simulink model "model"  (R2022b)
settings: Solver=VariableStepAuto  StartTime=0.0  StopTime=10.0  RelTol=1e-3
values from neighbouring files (symbols this model uses):
  A = [-4.979 0 0.036 3.01 ... (first row only)    [matricies.m]
  B = [8.584 ... (first row only)    [matricies.m]
undefined symbols (not defined in the file or in its folder): Humusoft, kalmf, MF624
libraries: sldrtlib x3, simulink x1
settings Model: Creator=efrem  LastModifiedBy=126893
settings DebuggingCC: UnconnectedInputMsg=warning  UnconnectedOutputMsg=warning  UnconnectedLineMsg=warning
settings ModelReferenceCC: EnableRefExpFcnMdlSchedulingChecks=on
settings RTWCC: DLArmComputeVersion=19.05

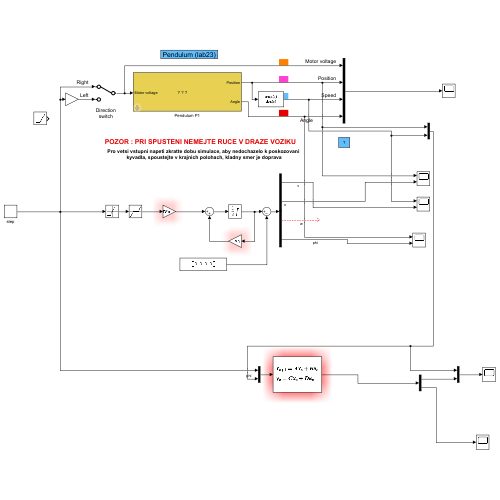
[thumbnail: Simulink's stored preview of the top-level diagram]
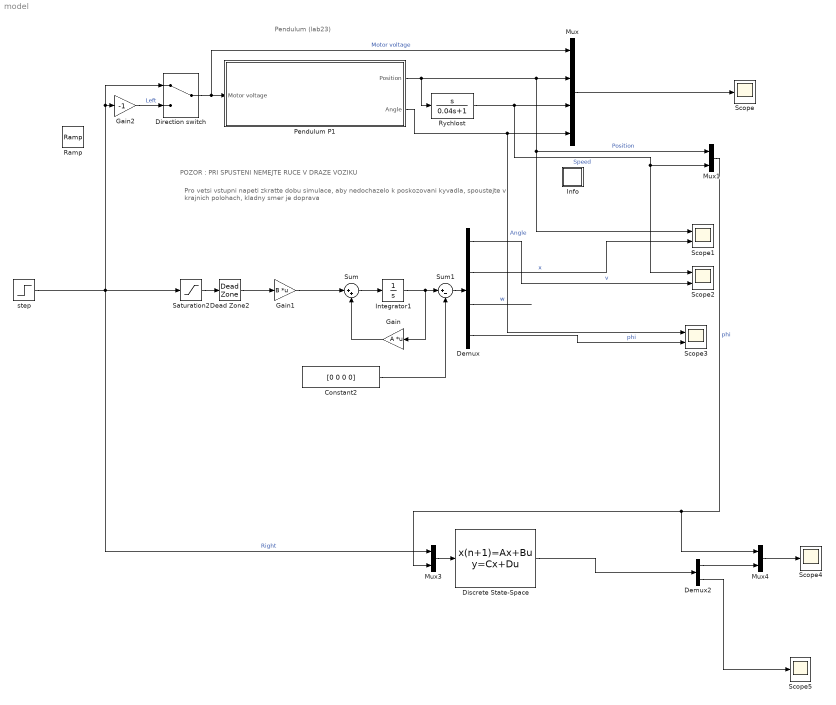
== system model ==
  note: POZOR : PRI SPUSTENI NEMEJTE RUCE V DRAZE VOZIKU
  note: Pro vetsi vstupni napeti zkratte dobu simulace, aby nedochazelo k poskozovani
      |  kyvadla, spoustejte v krajnich polohach, kladny smer je doprava
  note: Pendulum (lab23)
  Constant2 : Constant  Value=[0 0 0 0]
  Dead Zone2 : DeadZone  LowerValue=-0.11  UpperValue=0.11
  Demux : Demux
      settings: DisplayOption=none
  Demux2 : Demux  Outputs=[1,2]
  Direction switch : ManualSwitch
  Discrete State-Space : DiscreteStateSpace  A=kalmf.A  B=kalmf.B  C=kalmf.C  D=kalmf.D  InitialCondition=[0.2,0]  SampleTime=kalmf.Ts
  Gain : Gain  Gain=A  Multiplication=Matrix(K*u)
  Gain1 : Gain  Gain=B  Multiplication=Matrix(K*u)
  Gain2 : Gain  Gain=-1
  Info : Subsystem
      mask Display: disp('?')
  Integrator1 : Integrator  InitialCondition=[0,0,0,0]  LimitOutput=on  UpperSaturationLimit=[inf, 0.35, inf, inf]  LowerSaturationLimit=-[inf, 0.35, inf, inf]
  Mux : Mux
  Mux1 : Mux  Inputs=2
  Mux3 : Mux  Inputs=2
  Mux4 : Mux  Inputs=2
  Pendulum P1 : Subsystem  InitFcn=warning off;  mask(Pendulum P1 in laboratory K23){Ts=0.001}
      mask prompts: Ts "Sampling time  {Ts = 0.001 s;   0.001 - 0.01 s}"
      mask help: Pendulum P1 in laboratory K23 - Real Time Communication
      mask Help:
      | Servo AMIRA S1, S4 in laboratory K23, K26 - Real Time Communication. <br><br>
      | 
      | This is a model of the Servomechanism, which is composed of two identical motors (motor and generator) connected together with solid motor shaft. First motor is used as a generator - it can be used to simulation of a varying  moment of inertia. The second motor takes control of the rotational speed of the servomechanism or the angle of turning of the motor shaft.<br>
      | 
      | There are two inputs and three outputs in the model. Inputs are voltages of generator and motor.
      | Outputs are speed of the servomechanism, the angle of turning of the motor shaft and current of the motor.<br><br>
      | In Simulink, the signals are normalized.
      mask Display: image(imread('P1pic.tif'))
  Ramp : simulink/Sources/Ramp  slope=1  start=0  InitialOutput=0
  Rychlost : TransferFcn  Numerator=[1 0]  Denominator=[0.04 1]
  Saturation2 : Saturate  UpperLimit=1  LowerLimit=-1
  Scope : Scope
  Scope1 : Scope  NumInputPorts=2
  Scope2 : Scope  NumInputPorts=2
  Scope3 : Scope  NumInputPorts=2
  Scope4 : Scope
  Scope5 : Scope
  Sum : Sum  Inputs=|++
  Sum1 : Sum  Inputs=|+-
  step : Step  After=0.2  SampleTime=0
  wires:
  Gain1/1 -> Sum/1
  Dead Zone2/1 -> Gain1/1
  Sum/1 -> Integrator1/1
  Gain/1 -> Sum/2
  Demux/2 -> Scope1/2  "x"
  Demux/1 -> Scope2/2  "v"
  Integrator1/1 -> Gain/1, Sum1/1
  Saturation2/1 -> Dead Zone2/1
  Sum1/1 -> Demux/1
  Constant2/1 -> Sum1/2
  Demux/3 -> ?  "w"
  Demux/4 -> Scope3/2  "phi"
  Direction switch/1 -> Pendulum P1/1(Motor voltage), Mux/1  "Motor voltage"
  Rychlost/1 -> Mux1/2, Scope2/1, Mux/3  "Speed"
  Pendulum P1/2(Angle) -> Scope3/1, Mux/4  "Angle"
  Gain2/1 -> Direction switch/2  "Left"
  Pendulum P1/1(Position) -> Scope1/1, Mux1/1, Mux/2, Rychlost/1  "Position"
  step/1 -> Saturation2/1, Mux3/1, Direction switch/1, Gain2/1  "Right"
  Mux/1 -> Scope/1
  Demux2/1 -> Mux4/2
  Discrete State-Space/1 -> Demux2/1
  Demux2/2 -> Scope5/1
  Mux4/1 -> Scope4/1
  Mux3/1 -> Discrete State-Space/1
  Mux1/1 -> Mux4/1, Mux3/2  "phi"

== system model/Info ==
  note: Urceno pro mereni prechodovych charakteristik realneho systemu inverzni kyvadlo.
      |  Periodu vzorkovani Ts volte v rozsahu 0.0005 s < Ts < 0.001 s  (dop. Ts = 0.001 s).
  note: Vozik presunte do leve krajni polohy. Po spusteni simulace dojede k prave krajni
      | poloze. Presunte jej ke koncovemu spinaci a zmente znamenko zesileni. Vozik
      | se vrati do vychozi polohy. Pri vetsim vstupnim napeti zkratte dobu simulace!!!
  note: Umisteni voziku
  note: Merena data jsou ukladana po radcich do matice ty v pracovnim prostoru Matlabu.
      | Prvni sloupec matice ty predstavuje cas a dalsi pak jednotlive promenne v poradi
      | vstupu do bloku multiplexoru osciloskopu. Krome toho je jeste k dispozici samotny
      | vektor casu tout. Prubehy velicin zobrazite napr. prikazem: plot(ty(:,1),ty(:,2:4)).
  note: Nezapomente si ulozit namerena data napr. prikazem: save <jmeno> ty
  note: Ve formatu ASCII je pak ulozite prikazem: save <jmeno> ty -ascii
  note: C: J.Fuka 2007-2015 pro Matlab 2014b s RTWT
  note: Kyvadlo P1 (lab. 23)

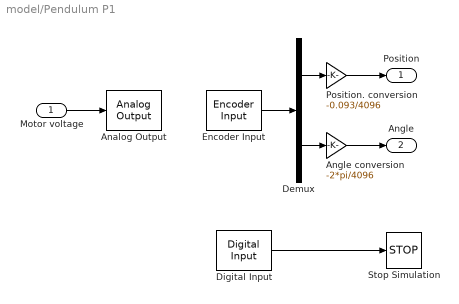
== system model/Pendulum P1 ==
  Motor voltage : Inport
  Analog Output : sldrtlib/Analog Output  SampleTime=Ts  MaxMissedTicks=200  ShowMissedTicks=off  YieldWhenWaiting=on  DrvName=Humusoft/MF624  DrvAddress=4294967295  DrvOptions=0  Channels=1  RangeMode=2  VoltRange=1  InitialValue=0  FinalValue=0
      settings: AttributesFormatString=Humusoft\nMF624 [auto]
  Angle conversion : Gain  Gain=-2*pi/4096
  Demux : Demux  Outputs=2
      settings: DisplayOption=none
  Digital Input : sldrtlib/Digital Input  SampleTime=0.005  MaxMissedTicks=100  ShowMissedTicks=off  YieldWhenWaiting=off  DrvName=Humusoft/MF624  DrvAddress=4294967295  DrvOptions=0  Channels=3  BitMode=1  DataType=9
      settings: AttributesFormatString=Humusoft\nMF624 [auto]
  Encoder Input : sldrtlib/Encoder Input  SampleTime=Ts  MaxMissedTicks=200  ShowMissedTicks=off  YieldWhenWaiting=on  DrvName=Humusoft/MF624  DrvAddress=4294967295  DrvOptions=0  Channels=[1 2]  QuadMode=3  IndexPulse=2  InputFilter=Inf  DataType=1
      settings: AttributesFormatString=Humusoft\nMF624 [auto]
  Position. conversion : Gain  Gain=-0.093/4096
  Stop Simulation : Stop
  Position : Outport
  Angle : Outport  Port=2
  wires:
  Position. conversion/1 -> Position/1
  Demux/2 -> Angle conversion/1
  Angle conversion/1 -> Angle/1
  Encoder Input/1 -> Demux/1
  Demux/1 -> Position. conversion/1
  Digital Input/1 -> Stop Simulation/1
  Motor voltage/1 -> Analog Output/1
